simulink model "integrator"  (Simulink 4.00)
settings: Solver=ode45  StartTime=0.0  StopTime=tfinal  MaxStep=0.01  RelTol=1e-3
settings Model: LastModifiedBy=rajamani  OutputOption=SpecifiedOutputTimes  OutputTimes=t

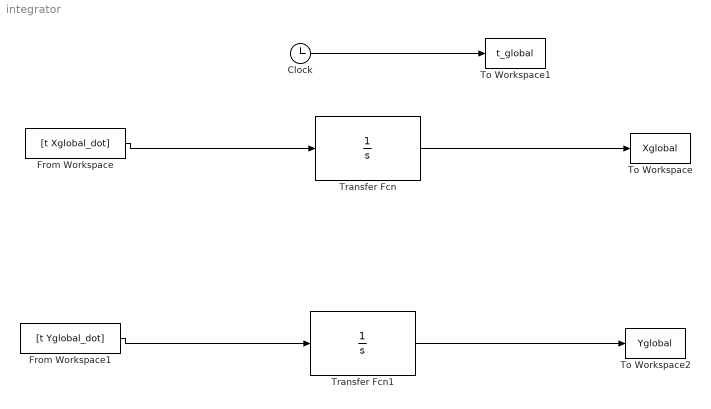
== system integrator ==
  Clock : Clock
      settings: DisplayTime=off  Decimation=10
  From Workspace : FromWorkspace  VariableName=[t Xglobal_dot]  SampleTime=0  OutputAfterFinalValue=Extrapolation
  From Workspace1 : FromWorkspace  VariableName=[t Yglobal_dot]  SampleTime=0  OutputAfterFinalValue=Extrapolation
  To Workspace : ToWorkspace  VariableName=Xglobal  SampleTime=-1  SaveFormat=Array
  To Workspace1 : ToWorkspace  VariableName=t_global  SampleTime=-1  SaveFormat=Array
  To Workspace2 : ToWorkspace  VariableName=Yglobal  SampleTime=-1  SaveFormat=Array
  Transfer Fcn : TransferFcn  Numerator=[1]  Denominator=[1 0]  AbsoluteTolerance=auto  Realization=auto
  Transfer Fcn1 : TransferFcn  Numerator=[1]  Denominator=[1 0]  AbsoluteTolerance=auto  Realization=auto
  wires:
  From Workspace/1 -> Transfer Fcn/1
  Transfer Fcn/1 -> To Workspace/1
  Clock/1 -> To Workspace1/1
  From Workspace1/1 -> Transfer Fcn1/1
  Transfer Fcn1/1 -> To Workspace2/1
